simulink model "Second"  (R2018a)
settings: Solver=FixedStepDiscrete  StartTime=0.0  StopTime=8  FixedStep=1  RelTol=1e-3
libraries: simulink x1
settings Model: Creator=Eng_Omar  LastModifiedBy=Eng_Omar
settings SolverCC: AutoInsertRateTranBlk=on
settings OptimizationCC: DefaultParameterBehavior=Inlined  EnhancedBackFolding=on  PassReuseOutputArgsAs=Individual arguments  MaxStackSize=64  OptimizeBlockOrder=speed  DifferentSizesBufferReuse=on  OptimizationCustomize=off
settings DebuggingCC: ParameterTunabilityLossMsg=error
settings SFSimCC: MATLABDynamicMemAlloc=off
settings RTWCC: SystemTargetFile=ert.tlc  GenCodeOnly=on  TemplateMakefile=ert_default_tmf  GenerateReport=on  Toolchain=Catkin  IncludeHyperlinkInReport=on  LaunchReport=on  GenerateTraceInfo=on  GenerateTraceReport=on  GenerateTraceReportSl=on  GenerateTraceReportSf=on  GenerateTraceReportEml=on
settings CodeAppCC: ForceParamTrailComments=on  IgnoreCustomStorageClasses=off  OperatorAnnotations=on  SimulinkDataObjDesc=on  SFDataObjDesc=on  InsertBlockDesc=on
settings ERTTargetCC: GenerateSampleERTMain=on  MultiInstanceERTCode=on  CodeInterfacePackaging=Reusable function  InlinedParameterPlacement=NonHierarchical  ERTCustomFileTemplate=example_file_process.tlc

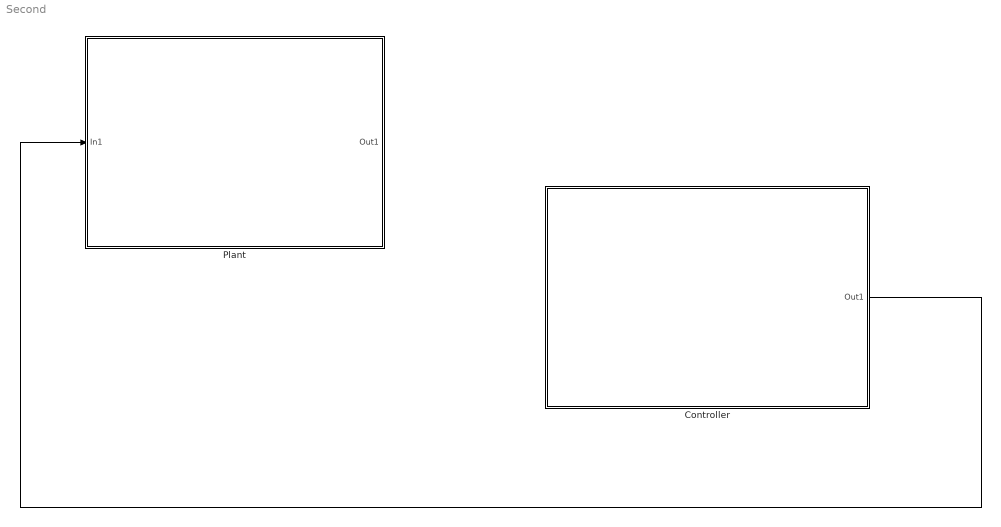
== system Second ==
  "Controller " : Subsystem
  "Plant " : Subsystem
  wires:
  "Controller "/1(Out1) -> "Plant "/1(In1)

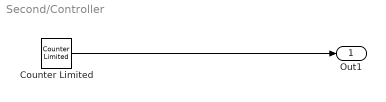
== system Second/Controller  ==
  Counter Limited : simulink/Sources/Counter Limited  uplimit=9  tsamp=-1
  Out1 : Outport
  wires:
  Counter Limited/1 -> Out1/1

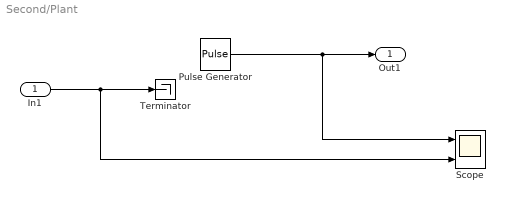
== system Second/Plant  ==
  In1 : Inport
  Pulse Generator : DiscretePulseGenerator  Amplitude=5  Period=1
  Scope : Scope  NumInputPorts=2
  Terminator : Terminator
  Out1 : Outport
  wires:
  In1/1 -> Scope/2, Terminator/1
  Pulse Generator/1 -> Scope/1, Out1/1
